simulink model "gm_PmodACL_IP_14a"  (R2014b)
settings: Solver=FixedStepDiscrete  StartTime=0.0  StopTime=4000  FixedStep=1  RelTol=1e-3
libraries: hdlsllib x11, simulink x4
settings Model: Creator=bsoheili  LastModifiedBy=dlwalter
settings DataIOCC: SaveOutput=off  SaveTime=off
settings OptimizationCC: BlockReduction=off  ConditionallyExecuteInputs=off  InlineParams=on  UseDivisionForNetSlopeComputation=UseDivisionForReciprocalsOfIntegersOnly  UseFloatMulNetSlope=on  InlineInvariantSignals=on  EnhancedBackFolding=on  EfficientFloat2IntCast=on  OptimizeModelRefInitCode=on  LifeSpan=1
settings DebuggingCC: AlgebraicLoopMsg=error  InheritedTsInSrcMsg=none  StrictBusMsg=ErrorOnBusTreatedAsVector  NonBusSignalsTreatedAsBus=error
settings HardwareCC: ProdHWDeviceType=ASIC/FPGA->ASIC/FPGA  ProdEqTarget=off
settings RTWCC: SystemTargetFile=ert.tlc  TemplateMakefile=ert_default_tmf  Description=Embedded Coder  GenerateReport=on  ProcessScript=ert_make_rtw_hook  IncludeHyperlinkInReport=on  LaunchReport=on  GenerateTraceInfo=on  GenerateTraceReport=on  GenerateTraceReportSl=on  GenerateTraceReportSf=on  GenerateTraceReportEml=on  GenerateCodeMetricsReport=on
settings CodeAppCC: IgnoreCustomStorageClasses=off
settings ERTTargetCC: GenerateSampleERTMain=on  CombineSignalStateStructs=on  SuppressErrorStatus=on  InlinedParameterPlacement=NonHierarchical  ERTCustomFileTemplate=example_file_process.tlc

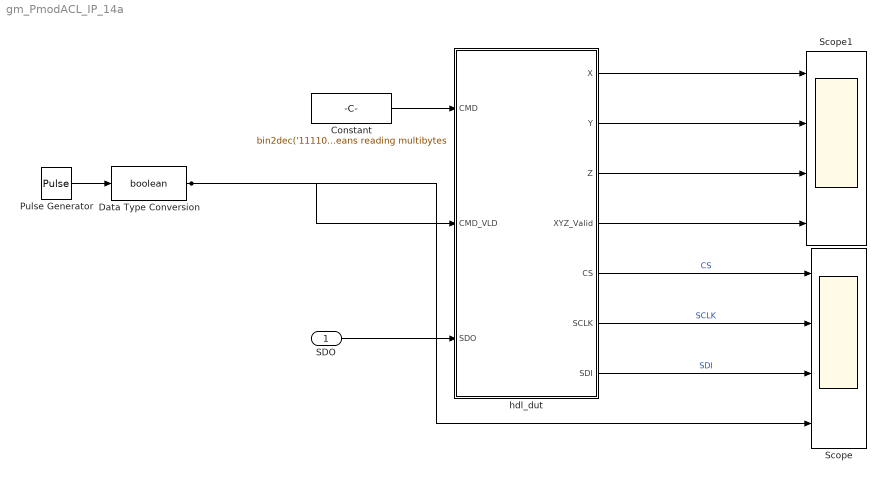
== system gm_PmodACL_IP_14a ==
  SDO : Inport  OutDataTypeStr=boolean
  Constant : Constant  Value="bin2dec('1111001100110011')  % 11 in msb means reading multibytes"  OutDataTypeStr=fixdt(0,16,0)  SampleTime=-1
  Data Type Conversion : DataTypeConversion  OutDataTypeStr=boolean
  Pulse Generator : DiscretePulseGenerator  Period=500  PhaseDelay=53
  Scope : Scope  NumInputPorts=4
      settings: TickLabels=on  TimeRange=2000  YMin=-5~-5~-5~-5  YMax=5~5~5~5
  Scope1 : Scope  NumInputPorts=4
      settings: TickLabels=on  TimeRange=2000  YMin=-5~-5~-5~-5  YMax=5~5~5~5  SaveName=ScopeData2
  hdl_dut : Subsystem  TreatAsAtomicUnit=on
  wires:
  hdl_dut/4(XYZ_Valid) -> Scope1/4
  Constant/1 -> hdl_dut/1(CMD)
  Pulse Generator/1 -> Data Type Conversion/1
  hdl_dut/7(SDI) -> Scope/3  "SDI"
  hdl_dut/6(SCLK) -> Scope/2  "SCLK"
  hdl_dut/5(CS) -> Scope/1  "CS"
  hdl_dut/3(Z) -> Scope1/3
  hdl_dut/2(Y) -> Scope1/2
  hdl_dut/1(X) -> Scope1/1
  SDO/1 -> hdl_dut/3(SDO)
  Data Type Conversion/1 -> hdl_dut/2(CMD_VLD), Scope/4

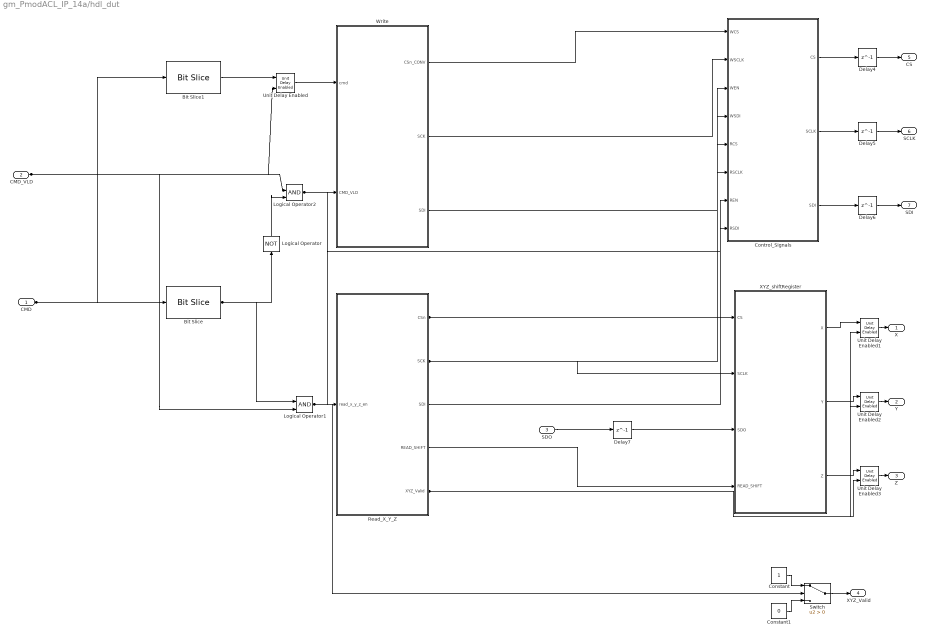
== system gm_PmodACL_IP_14a/hdl_dut ==
  CMD : Inport
  CMD_VLD : Inport  Port=2
  SDO : Inport  Port=3
  Bit Slice : hdlsllib/HDL Operations/Bit Slice  lidx=15  ridx=15
  Bit Slice1 : hdlsllib/HDL Operations/Bit Slice  lidx=13  ridx=0
  Constant : Constant  OutDataTypeStr=boolean
  Constant1 : Constant  Value=0  OutDataTypeStr=boolean
  Control_Signals : Subsystem
  Delay{4..7} (4 alike) : Delay  DelayLength=1  InitialCondition=0
  Logical Operator : Logic  Operator=NOT  IconShape=distinctive  AllPortsSameDT=off  OutDataTypeStr=boolean
  Logical Operator1 : Logic  IconShape=distinctive  AllPortsSameDT=off  OutDataTypeStr=boolean
  Logical Operator2 : Logic  IconShape=distinctive  AllPortsSameDT=off  OutDataTypeStr=boolean
  Read_X_Y_Z : Subsystem
  Switch : Switch  Criteria=u2 > Threshold
  Unit Delay Enabled{,1..3} (4 alike) : simulink/Additional Math & Discrete/Additional Discrete/Unit Delay Enabled  vinit=0.0  tsamp=-1
  Write : Subsystem
  XYZ_shiftRegister : Subsystem
  X : Outport
  Y : Outport  Port=2
  Z : Outport  Port=3
  XYZ_Valid : Outport  Port=4
  CS : Outport  Port=5
  SCLK : Outport  Port=6
  SDI : Outport  Port=7
  wires:
  CMD/1 -> Bit Slice1/1, Bit Slice/1
  CMD_VLD/1 -> Logical Operator2/1, Logical Operator1/2, Unit Delay Enabled/2
  SDO/1 -> Delay7/1
  Bit Slice/1 -> Logical Operator1/1, Logical Operator/1
  Bit Slice1/1 -> Unit Delay Enabled/1
  Constant/1 -> Switch/1
  Constant1/1 -> Switch/3
  Control_Signals/1(CS) -> Delay4/1
  Control_Signals/2(SCLK) -> Delay5/1
  Control_Signals/3(SDI) -> Delay6/1
  Delay4/1 -> CS/1
  Delay5/1 -> SCLK/1
  Delay6/1 -> SDI/1
  Delay7/1 -> XYZ_shiftRegister/3(SDO)
  Logical Operator/1 -> Logical Operator2/2
  Logical Operator1/1 -> Switch/2, Read_X_Y_Z/1(read_x_y_z_en), Control_Signals/7(REN)
  Logical Operator2/1 -> Write/2(CMD_VLD), Control_Signals/3(WEN)
  Read_X_Y_Z/1(CSn) -> Control_Signals/5(RCS), XYZ_shiftRegister/1(CS)
  Read_X_Y_Z/2(SCK) -> Control_Signals/6(RSCLK), XYZ_shiftRegister/2(SCLK)
  Read_X_Y_Z/3(SDI) -> Control_Signals/8(RSDI)
  Read_X_Y_Z/4(READ_SHIFT) -> XYZ_shiftRegister/4(READ_SHIFT)
  Read_X_Y_Z/5(XYZ_Valid) -> Unit Delay Enabled3/2, Unit Delay Enabled2/2, Unit Delay Enabled1/2
  Switch/1 -> XYZ_Valid/1
  Unit Delay Enabled/1 -> Write/1(cmd)
  Unit Delay Enabled1/1 -> X/1
  Unit Delay Enabled2/1 -> Y/1
  Unit Delay Enabled3/1 -> Z/1
  Write/1(CSn_CONV) -> Control_Signals/1(WCS)
  Write/2(SCK) -> Control_Signals/2(WSCLK)
  Write/3(SDI) -> Control_Signals/4(WSDI)
  XYZ_shiftRegister/1(X) -> Unit Delay Enabled1/1
  XYZ_shiftRegister/2(Y) -> Unit Delay Enabled2/1
  XYZ_shiftRegister/3(Z) -> Unit Delay Enabled3/1

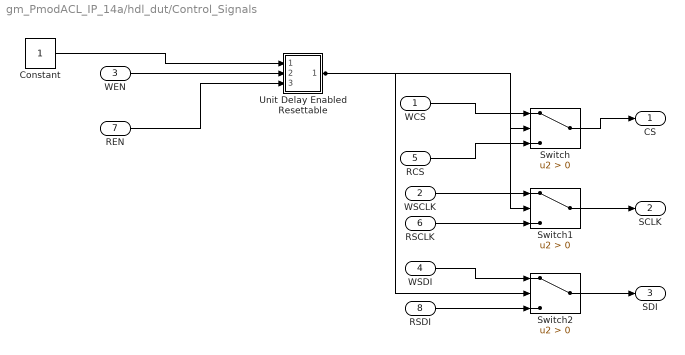
== system gm_PmodACL_IP_14a/hdl_dut/Control_Signals ==
  WCS : Inport
  WSCLK : Inport  Port=2
  WEN : Inport  Port=3
  WSDI : Inport  Port=4
  RCS : Inport  Port=5
  RSCLK : Inport  Port=6
  REN : Inport  Port=7
  RSDI : Inport  Port=8
  Constant : Constant  OutDataTypeStr=boolean  SampleTime=-1
  Switch : Switch  Criteria=u2 > Threshold
  Switch1 : Switch  Criteria=u2 > Threshold
  Switch2 : Switch  Criteria=u2 > Threshold
  Unit Delay Enabled Resettable : Subsystem
  CS : Outport
  SCLK : Outport  Port=2
  SDI : Outport  Port=3
  wires:
  WCS/1 -> Switch/1
  WSCLK/1 -> Switch1/1
  WEN/1 -> Unit Delay Enabled Resettable/2(Enb)
  WSDI/1 -> Switch2/1
  RCS/1 -> Switch/3
  RSCLK/1 -> Switch1/3
  REN/1 -> Unit Delay Enabled Resettable/3(Reset)
  RSDI/1 -> Switch2/3
  Constant/1 -> Unit Delay Enabled Resettable/1(data_in)
  Switch/1 -> CS/1
  Switch1/1 -> SCLK/1
  Switch2/1 -> SDI/1
  Unit Delay Enabled Resettable/1(data_out) -> Switch2/2, Switch1/2, Switch/2

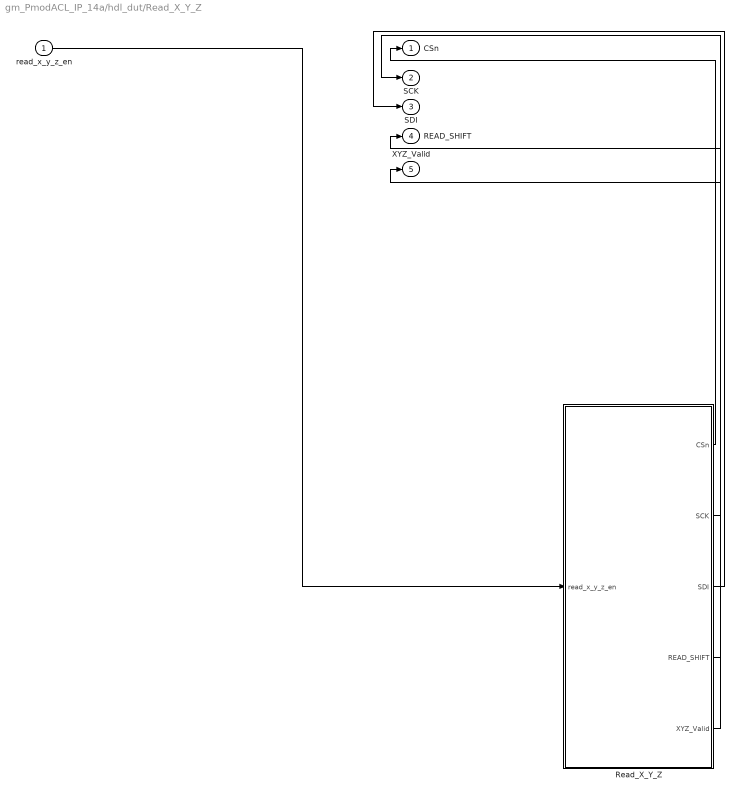
== system gm_PmodACL_IP_14a/hdl_dut/Read_X_Y_Z ==
  read_x_y_z_en : Inport
  Read_X_Y_Z : Stateflow chart  TreatAsAtomicUnit=on
  CSn : Outport
  SCK : Outport  Port=2
  SDI : Outport  Port=3
  READ_SHIFT : Outport  Port=4
  XYZ_Valid : Outport  Port=5
  wires:
  read_x_y_z_en/1 -> Read_X_Y_Z/1(read_x_y_z_en)
  Read_X_Y_Z/1(CSn) -> CSn/1
  Read_X_Y_Z/2(SCK) -> SCK/1
  Read_X_Y_Z/3(SDI) -> SDI/1
  Read_X_Y_Z/4(READ_SHIFT) -> READ_SHIFT/1
  Read_X_Y_Z/5(XYZ_Valid) -> XYZ_Valid/1

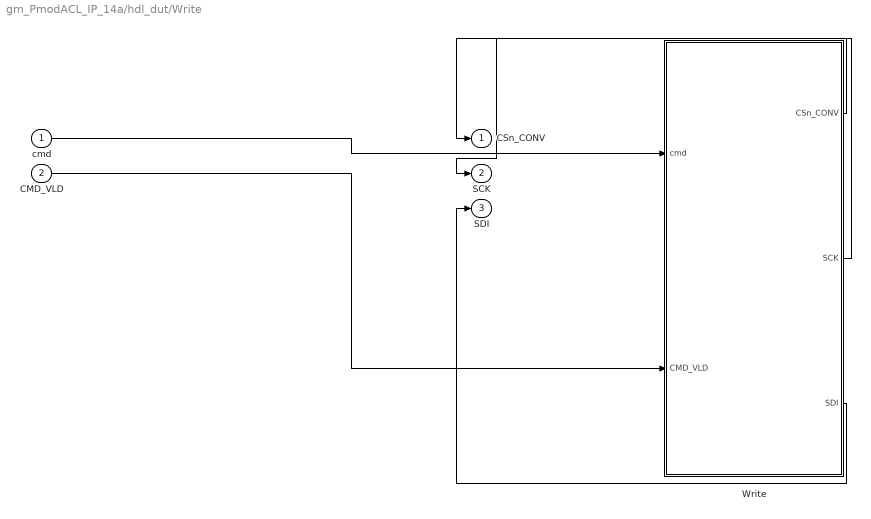
== system gm_PmodACL_IP_14a/hdl_dut/Write ==
  cmd : Inport
  CMD_VLD : Inport  Port=2
  Write : Stateflow chart  TreatAsAtomicUnit=on
  CSn_CONV : Outport
  SCK : Outport  Port=2
  SDI : Outport  Port=3
  wires:
  cmd/1 -> Write/1(cmd)
  CMD_VLD/1 -> Write/2(CMD_VLD)
  Write/1(CSn_CONV) -> CSn_CONV/1
  Write/2(SCK) -> SCK/1
  Write/3(SDI) -> SDI/1

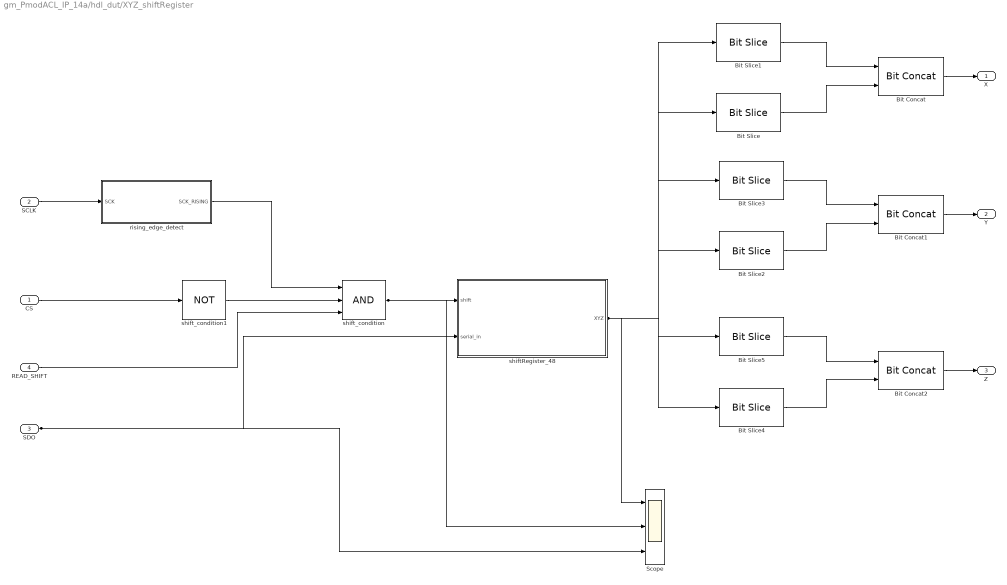
== system gm_PmodACL_IP_14a/hdl_dut/XYZ_shiftRegister ==
  CS : Inport
  SCLK : Inport  Port=2
  SDO : Inport  Port=3
  READ_SHIFT : Inport  Port=4
  Bit Concat : hdlsllib/HDL Operations/Bit Concat  numInputs=2
  Bit Concat1 : hdlsllib/HDL Operations/Bit Concat  numInputs=2
  Bit Concat2 : hdlsllib/HDL Operations/Bit Concat  numInputs=2
  Bit Slice : hdlsllib/HDL Operations/Bit Slice  lidx=47  ridx=40
  Bit Slice1 : hdlsllib/HDL Operations/Bit Slice  lidx=39  ridx=32
  Bit Slice2 : hdlsllib/HDL Operations/Bit Slice  lidx=31  ridx=24
  Bit Slice3 : hdlsllib/HDL Operations/Bit Slice  lidx=23  ridx=16
  Bit Slice4 : hdlsllib/HDL Operations/Bit Slice  lidx=15  ridx=8
  Bit Slice5 : hdlsllib/HDL Operations/Bit Slice  lidx=7  ridx=0
  Scope : Scope  NumInputPorts=3
      settings: TickLabels=on  YMin=-5~-5~-5  YMax=5~5~5  SaveName=ScopeData3
  rising_edge_detect : Subsystem
  shiftRegister_48 : Subsystem
  shift_condition : Logic  Inputs=3  IconShape=distinctive  AllPortsSameDT=off  OutDataTypeStr=boolean
  shift_condition1 : Logic  Operator=NOT  Inputs=3  IconShape=distinctive  AllPortsSameDT=off  OutDataTypeStr=boolean
  X : Outport
  Y : Outport  Port=2
  Z : Outport  Port=3
  wires:
  CS/1 -> shift_condition1/1
  SCLK/1 -> rising_edge_detect/1(SCK)
  SDO/1 -> Scope/3, shiftRegister_48/2(serial_in)
  READ_SHIFT/1 -> shift_condition/3
  Bit Concat/1 -> X/1
  Bit Concat1/1 -> Y/1
  Bit Concat2/1 -> Z/1
  Bit Slice/1 -> Bit Concat/2
  Bit Slice1/1 -> Bit Concat/1
  Bit Slice2/1 -> Bit Concat1/2
  Bit Slice3/1 -> Bit Concat1/1
  Bit Slice4/1 -> Bit Concat2/2
  Bit Slice5/1 -> Bit Concat2/1
  rising_edge_detect/1(SCK_RISING) -> shift_condition/1
  shiftRegister_48/1(XYZ) -> Bit Slice5/1, Bit Slice4/1, Bit Slice3/1, Bit Slice2/1, Bit Slice1/1, Bit Slice/1, Scope/1
  shift_condition/1 -> Scope/2, shiftRegister_48/1(shift)
  shift_condition1/1 -> shift_condition/2

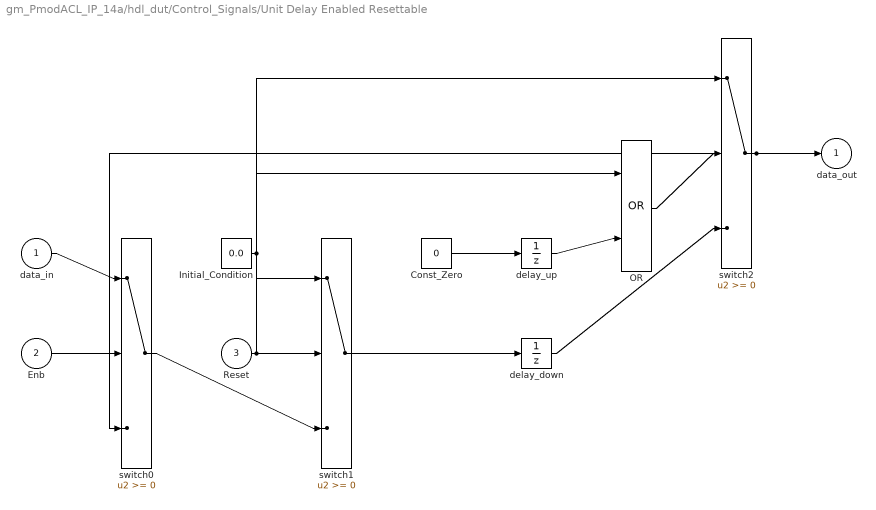
== system gm_PmodACL_IP_14a/hdl_dut/Control_Signals/Unit Delay Enabled Resettable ==
  data_in : Inport
  Enb : Inport  Port=2
  Reset : Inport  Port=3
  Const_Zero : Constant  Value=0  OutDataTypeStr=boolean
  Initial_Condition : Constant  Value=0.0  OutDataTypeStr=Inherit: Inherit via back propagation
  OR : Logic  Operator=OR
  delay_down : UnitDelay  SampleTime=-1
  delay_up : UnitDelay  InitialCondition=1  SampleTime=-1
  switch0 : Switch  SaturateOnIntegerOverflow=on  InputSameDT=on
  switch1 : Switch  SaturateOnIntegerOverflow=on  InputSameDT=on
  switch2 : Switch  SaturateOnIntegerOverflow=on  InputSameDT=on
  data_out : Outport
  wires:
  data_in/1 -> switch0/1
  Enb/1 -> switch0/2
  switch2/1 -> switch0/3, data_out/1
  Initial_Condition/1 -> switch1/1, switch2/1
  Reset/1 -> switch1/2, OR/1
  switch0/1 -> switch1/3
  Const_Zero/1 -> delay_up/1
  switch1/1 -> delay_down/1
  delay_up/1 -> OR/2
  OR/1 -> switch2/2
  delay_down/1 -> switch2/3

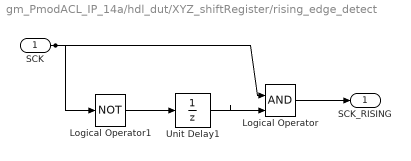
== system gm_PmodACL_IP_14a/hdl_dut/XYZ_shiftRegister/rising_edge_detect ==
  SCK : Inport
  Logical Operator : Logic  IconShape=distinctive  AllPortsSameDT=off  OutDataTypeStr=boolean
  Logical Operator1 : Logic  Operator=NOT  IconShape=distinctive  AllPortsSameDT=off  OutDataTypeStr=boolean
  Unit Delay1 : UnitDelay  SampleTime=-1
  SCK_RISING : Outport
  wires:
  SCK/1 -> Logical Operator1/1, Logical Operator/1
  Logical Operator/1 -> SCK_RISING/1
  Logical Operator1/1 -> Unit Delay1/1
  Unit Delay1/1 -> Logical Operator/2

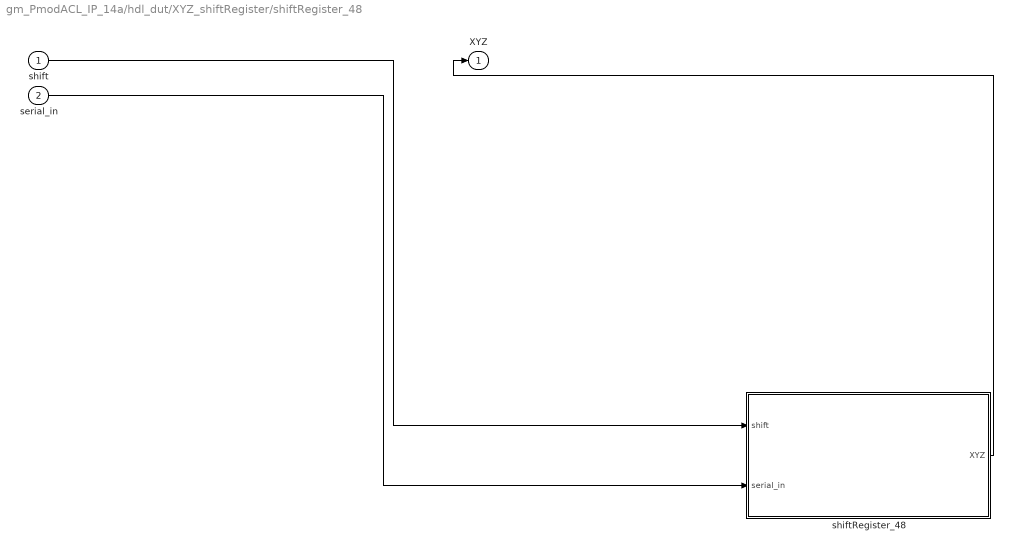
== system gm_PmodACL_IP_14a/hdl_dut/XYZ_shiftRegister/shiftRegister_48 ==
  shift : Inport
  serial_in : Inport  Port=2
  shiftRegister_48 : MATLAB Function  TreatAsAtomicUnit=on
  XYZ : Outport
  wires:
  shift/1 -> shiftRegister_48/1(shift)
  serial_in/1 -> shiftRegister_48/2(serial_in)
  shiftRegister_48/1(XYZ) -> XYZ/1

== matlab function gm_PmodACL_IP_14a/hdl_dut/XYZ_shiftRegister/shiftRegister_48/shiftRegister_48 ==
  data: shift input boolean; serial_in input; XYZ output fixdt(0,48,0)
function XYZ = fcn(shift, serial_in)
%#codegen

%%
persistent XYZ_int 
if isempty(XYZ_int)
    XYZ_int = fi(0,0,48,0);
end
%%


%%
if shift == true 
    serial_in_int = fi(serial_in, 0, 1, 0);
    XYZ_int = bitsll(XYZ_int, 1);
    XYZ_int = (bitconcat(bitsliceget(XYZ_int, 48, 2), serial_in_int));
end
%%
XYZ = XYZ_int;
%%

== stateflow chart gm_PmodACL_IP_14a/hdl_dut/Write/Write ==
  settings: executeAtInitialization=1
  note: This is single write to and address location. The write and MB bist
      | are hard coded. The 'cmd' is 14 bits. The upper 6 bits are address and
      | the lower 8 bits are data.
      | Here is the address map :
  state IDLE
  note: ?
  state START_CONV
    settings: description=|
        | During START_CONV the CSn_CONV is held high for 10 clock cycles.
        | Assuming the FPGA clock frequency is 100 MHz, the 10 clock count delay
        | provides 100 nS delay which is the typical time specified in the ADC data
        | sheet for the CSn_CONV input to the ADC.
        | 
        | The count comparator can be changed from 10 by the user as long as the ADC requirment for minimum of 40 nS is met.
  state tCONV_delay
    settings: description="tCoONV time is typical 3 uS and Maximum 3.5 uS according to ADC data sheet.  Assuming clock frequency of 100 MHz, the maximum count value for 3 uS delay should be (3 uS/10 nS=) 300."
  state START_ADC_RDWR
    settings: description="The ADC maximum clock frequency, according to ADC data sheet, is rated at 40 MHz.  Assuming a 100 MHz FPGA clock dividing the FPGA clock by 3 to generate a 33.33 MHz ADC clock (SCK) for the ADC."
  state CLOCKING
    settings: description="tCoONV time is typical 3 uS and Maximum 3.5 uS according to ADC data sheet.  Assuming clock frequency of 100 MHz, the maximum count value for 3 uS delay should be (3 uS/10 nS=) 300."
  state END1
  state END
  (default) -> IDLE
  END -> IDLE
  IDLE -> START_CONV : [CMD_VLD == true]{CSn_CONV = false;...
      | SCK = false;
      | SDI = false; } % sdi_gen(cmd ,clock_cnt);}
  START_CONV -> START_CONV [order 2] : {count++;}
  START_CONV -> tCONV_delay [order 1] : [count == 10]{count = 0; CSn_CONV = false; SCK = true;}
  tCONV_delay -> tCONV_delay [order 2] : {count++;}
  tCONV_delay -> START_ADC_RDWR [order 1] : [count ==10]...
      | {count = 0;
      | SCK = false;}
  CLOCKING -> CLOCKING [order 2] : {count++;}
  START_ADC_RDWR -> START_ADC_RDWR [order 3] : {count++;}
  START_ADC_RDWR -> CLOCKING [order 2] : [count == 10]{count = 0;SCK=true;clock_cnt++;}
  CLOCKING -> START_ADC_RDWR [order 1] : [count == 10]{count = 0;...
      | SCK=false;
      | SDI = sdi_gen(cmd,clock_cnt);}
  START_ADC_RDWR -> END1 [order 1] : [clock_cnt == 14  && count == 10]...
      | {clock_cnt = 0;...
      | count = 0;
      | SCK = true;}
  END1 -> END1 [order 2] : {count++;}
  END1 -> END [order 1] : [count == 10]{count = 0; CSn_CONV = true;}
  data: word function_input fixdt(0,14,0); cnt function_input fixdt(0,5,0); ser_data function_output boolean; CSn_CONV output boolean =true; count local fixdt(0,9,0) =0; SCK output boolean =true; clock_cnt local fixdt(0,5,0) =0; SDI output boolean =true; cmd input fixdt(0,14,0); CMD_VLD input boolean
  function ser_data = sdi_gen(word,cnt):
    | function ser_data = sdi_gen(word,cnt)
    | 
    | 
    | persistent ser_data_int;
    | if isempty(ser_data_int)
    |     ser_data_int = false;
    | end
    | 
    | 
    | if cnt == fi(1,0,5,0)
    |     ser_data_int = logical(bitget(word, 14));
    | elseif cnt == fi(2,0,5,0)
    |     ser_data_int = logical(bitget(word, 13));
    | elseif cnt == fi(3,0,5,0)
    |     ser_data_int = logical(bitget(word, 12));
    | elseif cnt == fi(4,0,5,0)
    |     ser_data_int = logical(bitget(word, 11));
    | elseif cnt == fi(5,0,5,0)
    |     ser_data_int = logical(bitget(word, 10));
    | elseif cnt == fi(6,0,5,0)
    |     ser_data_int = logical(bitget(word, 9));
    | elseif cnt == fi(7,0,5,0)
    |     ser_data_int = logical(bitget(word, 8));
    | elseif cnt == fi(8,0,5,0)
    |     ser_data_int = logical(bitget(word, 7));
    | elseif cnt == fi(9,0,5,0)
    |     ser_data_int = logical(bitget(word, 6));
    | elseif cnt == fi(10,0,5,0)
    |     ser_data_int = logical(bitget(word, 5));
    | elseif cnt == fi(11,0,5,0)
    |     ser_data_int = logical(bitget(word, 4));
    | elseif cnt == fi(12,0,5,0)
    |     ser_data_int = logical(bitget(word, 3));
    | elseif cnt == fi(13,0,5,0)
    |     ser_data_int = logical(bitget(word, 2));
    | elseif cnt == fi(14,0,5,0)
    |     ser_data_int = logical(bitget(word, 1));
    | else
    |     ser_data_int = false;
    | end
    | 
    | ser_data = ser_data_int;

== stateflow chart gm_PmodACL_IP_14a/hdl_dut/Read_X_Y_Z/Read_X_Y_Z ==
  settings: executeAtInitialization=1
  state IDLE
  note: This chart reads the six X, Y, Z registers from ADXL345 chip
      |
      | !!!!!! Under construction !!!!!!
  note: ?
  state START_CONV
    settings: description=|
        | During START_CONV the CSn_CONV is held high for 10 clock cycles.
        | Assuming the FPGA clock frequency is 100 MHz, the 10 clock count delay
        | provides 100 nS delay which is the typical time specified in the ADC data
        | sheet for the CSn_CONV input to the ADC.
        | 
        | The count comparator can be changed from 10 by the user as long as the ADC requirment for minimum of 40 nS is met.
  state tCONV_delay
    settings: description="tCoONV time is typical 3 uS and Maximum 3.5 uS according to ADC data sheet.  Assuming clock frequency of 100 MHz, the maximum count value for 3 uS delay should be (3 uS/10 nS=) 300."
  state START_ADC_RDWR
    settings: description="The ADC maximum clock frequency, according to ADC data sheet, is rated at 40 MHz.  Assuming a 100 MHz FPGA clock dividing the FPGA clock by 3 to generate a 33.33 MHz ADC clock (SCK) for the ADC."
  state CLOCKING
    settings: description="tCoONV time is typical 3 uS and Maximum 3.5 uS according to ADC data sheet.  Assuming clock frequency of 100 MHz, the maximum count value for 3 uS delay should be (3 uS/10 nS=) 300."
  state Read1
  state Read
  state END
  END -> IDLE [order 1] : [count == 10]...
      | {CSn = true;
      | count = 0;
      | XYZ_Valid = true;
      | READ_SHIFT = false;}
  (default) -> IDLE
  IDLE -> START_CONV : [read_x_y_z_en == true]{CSn = false;
      | clock_cnt++;
      | XYZ_Valid = false;}
  START_CONV -> START_CONV [order 2] : {count++;}
  START_CONV -> tCONV_delay [order 1] : [count == 10]{count = 0; SCK = false;
      |   SDI = sdi_gen(cmd, clock_cnt);} % sending Read bit
  tCONV_delay -> tCONV_delay [order 2] : {count++;}
  tCONV_delay -> START_ADC_RDWR [order 1] : [count ==10]...
      | {count = 0;
      | SCK = true;
      | clock_cnt++;}
  CLOCKING -> CLOCKING [order 2] : {count++;}
  START_ADC_RDWR -> START_ADC_RDWR [order 3] : {count++;}
  START_ADC_RDWR -> CLOCKING [order 2] : [count == 10]{count = 0;SCK= false; SDI = sdi_gen(cmd, clock_cnt);}
  CLOCKING -> START_ADC_RDWR [order 1] : [count == 10]{count = 0;...
      | SCK=true;
      | clock_cnt++;}
  START_ADC_RDWR -> Read [order 1] : [clock_cnt == 9  && count == 10]...
      | {count = 0;
      | SCK = false;
      | SDI = true;
      | READ_SHIFT = true;}
  Read1 -> Read1 [order 2] : {count++;}
  Read -> Read1 [order 2] : [count == 10]{SCK = true;count = 0; clock_cnt++;}
  Read -> Read [order 3] : {count++;}
  Read1 -> Read [order 1] : [count == 10]{SCK = false;count = 0;}
  Read -> END [order 1] : [count == 10 && clock_cnt == 56]...
      | {count = 0;
      | clock_cnt = 0;
      | SCK = true;}
  END -> END [order 2] : {count++;}
  data: word function_input uint8; cnt function_input fixdt(0,5,0); ser_data function_output boolean; read_x_y_z_en input boolean; CSn output boolean =true; count local fixdt(0,9,0) =0; SCK output boolean =true; clock_cnt local fixdt(0,6,0) =0; SDI output boolean =true; cmd constant uint8 =242; READ_SHIFT output boolean =false; XYZ_Valid output boolean =true
  function ser_data = sdi_gen(word,cnt):
    | function ser_data = sdi_gen(word,cnt)
    | 
    | 
    | persistent ser_data_int;
    | if isempty(ser_data_int)
    |     ser_data_int = false;
    | end
    | 
    | 
    | if cnt == fi(1,0,5,0)
    |     ser_data_int = logical(bitget(word, 8));
    | elseif cnt == fi(2,0,5,0)
    |     ser_data_int = logical(bitget(word, 7));
    | elseif cnt == fi(3,0,5,0)
    |     ser_data_int = logical(bitget(word, 6));
    | elseif cnt == fi(4,0,5,0)
    |     ser_data_int = logical(bitget(word, 5));
    | elseif cnt == fi(5,0,5,0)
    |     ser_data_int = logical(bitget(word, 4));
    | elseif cnt == fi(6,0,5,0)
    |     ser_data_int = logical(bitget(word, 3));
    | elseif cnt == fi(7,0,5,0)
    |     ser_data_int = logical(bitget(word, 2));
    | elseif cnt == fi(8,0,5,0)
    |     ser_data_int = logical(bitget(word, 1));
    | else
    |     ser_data_int = true;
    | end
    | 
    | ser_data = ser_data_int;
